simulink model "prystupalab7_si"  (R2023b)
settings: Solver=VariableStepAuto  StartTime=0.0  StopTime=10.0  RelTol=1e-3
values from neighbouring files (symbols this model uses):
  A1 = 6    [prystupalab7_1.m]
  A2 = 6    [prystupalab7_1.m]
  dfw1 = 0    [prystupalab7_1.m]
  dfw2 = 0.1*fwmax2    [prystupalab7_1.m]
  fw1 = 0.1*fwmax2    [prystupalab7_1.m]
  fw2 = tabFw2(i)    [prystupalab7_1.m]
  t0 = 5    [prystupalab7_1.m]
undefined symbols (not defined in the file or in its folder): a1, a2, H01, H02
settings Model: Creator=Adam  LastModifiedBy=Adam

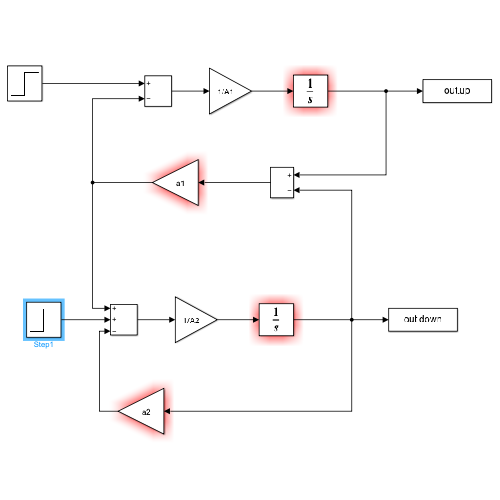
[thumbnail: Simulink's stored preview of the top-level diagram]
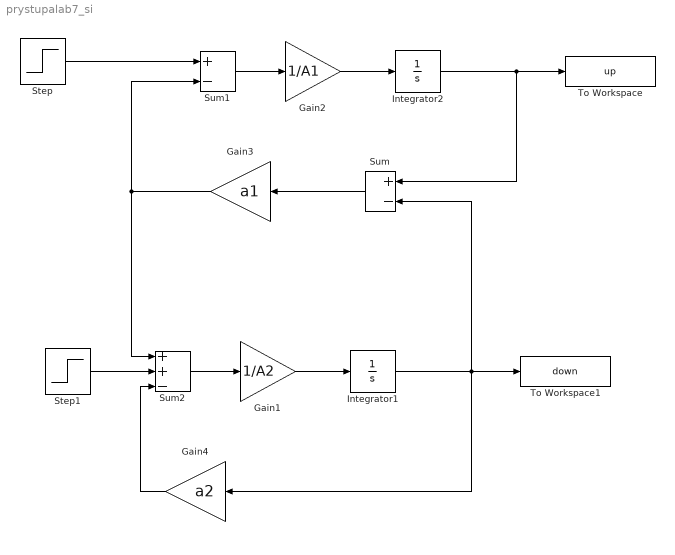
== system prystupalab7_si ==
  Gain1 : Gain  Gain=1/A2
  Gain2 : Gain  Gain=1/A1
  Gain3 : Gain  Gain=a1
  Gain4 : Gain  Gain=a2
  Integrator1 : Integrator  InitialCondition=H02
  Integrator2 : Integrator  InitialCondition=H01
  Step : Step  Time=t0  Before=fw1  After=fw1 + dfw1  SampleTime=0
  Step1 : Step  Time=t0  Before=fw2  After=fw2 + dfw2  SampleTime=0
  Sum : Sum  Inputs=+-
  Sum1 : Sum  Inputs=+-
  Sum2 : Sum  Inputs=++-
  To Workspace : ToWorkspace  VariableName=up  SampleTime=-1
  To Workspace1 : ToWorkspace  VariableName=down  SampleTime=-1
  wires:
  Sum1/1 -> Gain2/1
  Gain2/1 -> Integrator2/1
  Integrator2/1 -> Sum/1, To Workspace/1
  Step/1 -> Sum1/1
  Gain3/1 -> Sum2/1, Sum1/2
  Gain1/1 -> Integrator1/1
  Step1/1 -> Sum2/2
  Integrator1/1 -> Sum/2, To Workspace1/1, Gain4/1
  Gain4/1 -> Sum2/3
  Sum2/1 -> Gain1/1
  Sum/1 -> Gain3/1
